simulink model "DC_motor_impulseTest"  (R2013b)
settings: Solver=ode45  StartTime=0.0  StopTime=20  RelTol=1e-3
values from neighbouring files (symbols this model uses):
  J = 1.66e-5    (= 1.66e-05)    [RunMotorSim.m]    (also in RunMotorSim_OpenLoop.m)
  KD = 1.33e-8    (= 1.33e-08)    [RunMotorSim.m]    (also in RunMotorSim_OpenLoop.m)
  KT = 7.5e-3    (= 0.0075)    [RunMotorSim.m]    (also in RunMotorSim_OpenLoop.m)
  pow = 1.88    [RunMotorSim.m]    (also in RunMotorSim_OpenLoop.m = 2)
settings Model: Creator=aberger  LastModifiedBy=aberger

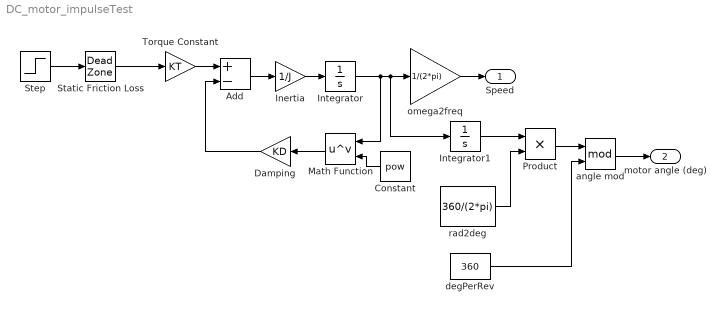
== system DC_motor_impulseTest ==
  Add : Sum  Inputs=+-
  Constant : Constant  Value=pow
  Damping : Gain  Gain=KD
  Inertia : Gain  Gain=1/J
  Integrator : Integrator
  Integrator1 : Integrator
  Math Function : Math  Operator=pow  SaturateOnIntegerOverflow=on
  Product : Product
  Static Friction Loss : DeadZone  LowerValue=-.05  UpperValue=.05  SaturateOnIntegerOverflow=on
  Step : Step  Time=0  After=0.1  SampleTime=0
  Torque Constant : Gain  Gain=KT
  angle mod : Math  Operator=mod  SaturateOnIntegerOverflow=on
  degPerRev : Constant  Value=360
  omega2freq : Gain  Gain=1/(2*pi)
  rad2deg : Constant  Value=360/(2*pi)
  Speed : Outport
  motor angle (deg) : Outport  Port=2
  wires:
  Add/1 -> Inertia/1
  Integrator/1 -> Math Function/1, Integrator1/1, omega2freq/1
  Torque Constant/1 -> Add/1
  Damping/1 -> Add/2
  Inertia/1 -> Integrator/1
  Step/1 -> Static Friction Loss/1
  Constant/1 -> Math Function/2
  Math Function/1 -> Damping/1
  omega2freq/1 -> Speed/1
  Integrator1/1 -> Product/1
  Product/1 -> angle mod/1
  rad2deg/1 -> Product/2
  degPerRev/1 -> angle mod/2
  Static Friction Loss/1 -> Torque Constant/1
  angle mod/1 -> motor angle (deg)/1
